simulink model "qrdrls_simulink"  (R2020b)
settings: Solver=FixedStepDiscrete  StartTime=0.0  StopTime=2000  RelTol=1e-3
libraries: dspsrcs4 x2
settings Model: MinMaxOverflowLogging=MinMaxAndOverflow  FPTRunName=NoOverride  Creator=andreas  LastModifiedBy=jgentile
settings DataIOCC: LimitDataPoints=on  SaveFormat=Array  InspectSignalLogs=on  ReturnWorkspaceOutputs=off
settings OptimizationCC: DefaultParameterBehavior=Inlined  ExpressionDepthLimit=2147483647  LifeSpan=inf  SimCompilerOptimization=on
settings DebuggingCC: SignalRangeChecking=warning  UnderspecifiedInitializationDetection=Classic  MergeDetectMultiDrivingBlocksExec=none  SolverPrmCheckMsg=warning  ParameterDowncastMsg=warning  ParameterOverflowMsg=warning  StateNameClashWarn=warning  StrictBusMsg=ErrorOnBusTreatedAsVector  SFUnexpectedBacktrackingDiag=warning  SFNoUnconditionalDefaultTransitionDiag=warning  SFExecutionAtInitializationDiag=none  ArithmeticOperatorsInVariantConditions=warning
settings HardwareCC: ProdBitPerPointer=32  ProdBitPerSizeT=32  ProdBitPerPtrDiffT=32  ProdLargestAtomicFloat=None  ProdIntDivRoundTo=Undefined  ProdEndianess=Unspecified  ProdWordSize=32  ProdHWDeviceType=Generic->Unspecified (assume 32-bit Generic)  TargetBitPerLong=64  TargetBitPerPointer=64  TargetBitPerSizeT=64  TargetBitPerPtrDiffT=64  TargetLongLongMode=on  TargetIntDivRoundTo=Zero  TargetEndianess=LittleEndian  TargetWordSize=64  TargetHWDeviceType=MATLAB Host  ProdEqTarget=off
settings ModelReferenceCC: EnableParallelModelReferenceBuilds=on  PropagateSignalLabelsOutOfModel=off
settings SFSimCC: SimUseLocalCustomCode=off  CustomCodeUndefinedFunction=UseInterfaceOnly
settings RTWCC: RTWUseLocalCustomCode=off
settings CodeAppCC: StateflowObjectComments=on
settings GRTTargetCC: TargetLangStandard=C89/C90 (ANSI)
settings ConfigComp: CovMetricSettings=dw  CovSaveCumulativeToWorkspaceVar=on  CovSaveSingleToWorkspaceVar=on  CovExternalEMLEnable=off

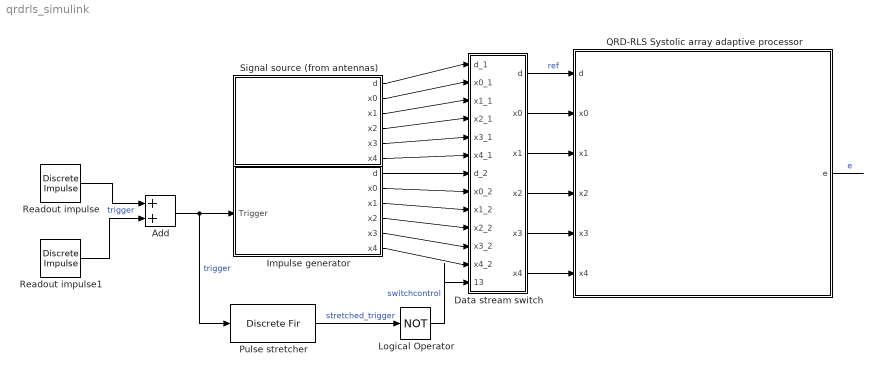
== system qrdrls_simulink ==
  Add : Sum
  Data stream switch : Subsystem
  Impulse generator : Subsystem
  Logical Operator : Logic  Operator=NOT  AllPortsSameDT=off  OutDataTypeStr=boolean
  Pulse stretcher : DiscreteFir  Coefficients=ones(1,6)
  QRD-RLS Systolic array adaptive processor : Subsystem
  Readout impulse : dspsrcs4/Discrete  Impulse  Delay=540  SampleTime=1  FrameSample=1  OutputFrames=on  dataType=double  isSigned=on  wordLen=16  udDataType=sfix(16)  fracBitsMode=Best precision  numFracBits=15  OutDataTypeStr=double  LastOutDataTypeStr=double
  Readout impulse1 : dspsrcs4/Discrete  Impulse  Delay=570  SampleTime=1  FrameSample=1  OutputFrames=on  dataType=double  isSigned=on  wordLen=16  udDataType=sfix(16)  fracBitsMode=Best precision  numFracBits=15  OutDataTypeStr=double  LastOutDataTypeStr=double
  Signal source (from antennas) : Subsystem
  wires:
  QRD-RLS Systolic array adaptive processor/1(e) -> ?  "e"
  Logical Operator/1 -> Data stream switch/13(selector)  "switchcontrol"
  Add/1 -> Pulse stretcher/1, Impulse generator/1(Trigger)  "trigger"
  Signal source (from antennas)/1(d) -> Data stream switch/1(d_1)
  Signal source (from antennas)/2(x0) -> Data stream switch/2(x0_1)
  Signal source (from antennas)/3(x1) -> Data stream switch/3(x1_1)
  Signal source (from antennas)/4(x2) -> Data stream switch/4(x2_1)
  Signal source (from antennas)/5(x3) -> Data stream switch/5(x3_1)
  Signal source (from antennas)/6(x4) -> Data stream switch/6(x4_1)
  Impulse generator/1(d) -> Data stream switch/7(d_2)
  Impulse generator/2(x0) -> Data stream switch/8(x0_2)
  Impulse generator/3(x1) -> Data stream switch/9(x1_2)
  Impulse generator/4(x2) -> Data stream switch/10(x2_2)
  Impulse generator/5(x3) -> Data stream switch/11(x3_2)
  Impulse generator/6(x4) -> Data stream switch/12(x4_2)
  Data stream switch/1(d) -> QRD-RLS Systolic array adaptive processor/1(d)  "ref"
  Data stream switch/2(x0) -> QRD-RLS Systolic array adaptive processor/2(x0)
  Data stream switch/3(x1) -> QRD-RLS Systolic array adaptive processor/3(x1)
  Data stream switch/4(x2) -> QRD-RLS Systolic array adaptive processor/4(x2)
  Data stream switch/5(x3) -> QRD-RLS Systolic array adaptive processor/5(x3)
  Data stream switch/6(x4) -> QRD-RLS Systolic array adaptive processor/6(x4)
  Pulse stretcher/1 -> Logical Operator/1  "stretched_trigger"
  Readout impulse/1 -> Add/1  "trigger"
  Readout impulse1/1 -> Add/2

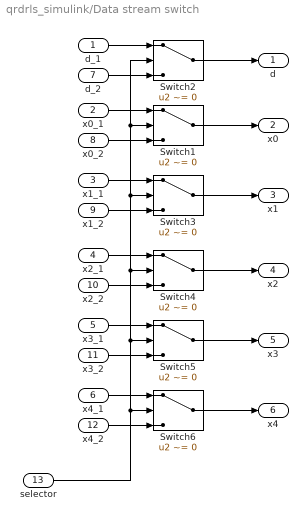
== system qrdrls_simulink/Data stream switch ==
  d_1 : Inport
  x0_1 : Inport  Port=2
  x1_1 : Inport  Port=3
  x2_1 : Inport  Port=4
  x3_1 : Inport  Port=5
  x4_1 : Inport  Port=6
  d_2 : Inport  Port=7
  x0_2 : Inport  Port=8
  x1_2 : Inport  Port=9
  x2_2 : Inport  Port=10
  x3_2 : Inport  Port=11
  x4_2 : Inport  Port=12
  selector : Inport  Port=13
  Switch{1..6} (6 alike) : Switch  Criteria=u2 ~= 0
  d : Outport
  x0 : Outport  Port=2
  x1 : Outport  Port=3
  x2 : Outport  Port=4
  x3 : Outport  Port=5
  x4 : Outport  Port=6
  wires:
  d_1/1 -> Switch2/1
  d_2/1 -> Switch2/3
  Switch2/1 -> d/1
  x0_1/1 -> Switch1/1
  x0_2/1 -> Switch1/3
  x1_1/1 -> Switch3/1
  x1_2/1 -> Switch3/3
  x2_1/1 -> Switch4/1
  x2_2/1 -> Switch4/3
  x3_1/1 -> Switch5/1
  x3_2/1 -> Switch5/3
  x4_1/1 -> Switch6/1
  x4_2/1 -> Switch6/3
  Switch1/1 -> x0/1
  Switch3/1 -> x1/1
  Switch4/1 -> x2/1
  Switch5/1 -> x3/1
  Switch6/1 -> x4/1
  selector/1 -> Switch6/2, Switch5/2, Switch4/2, Switch3/2, Switch1/2, Switch2/2

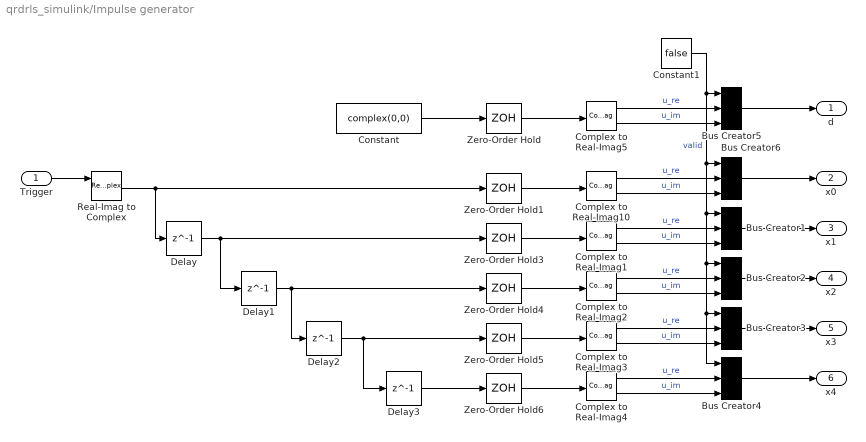
== system qrdrls_simulink/Impulse generator ==
  Trigger : Inport
  Bus Creator{1..6} (6 alike) : BusCreator  Inputs=3  OutDataTypeStr=Bus: vbus  NonVirtualBus=on
  Complex to Real-Imag{1..5,10} (6 alike) : ComplexToRealImag
  Constant : Constant  Value=complex(0,0)
  Constant1 : Constant  Value=false
  Delay{,1..3} (4 alike) : Delay  DelayLength=1  InitialCondition=0
  Real-Imag to Complex : RealImagToComplex
  Zero-Order Hold{,1,3..6} (6 alike) : ZeroOrderHold
  d : Outport
  x0 : Outport  Port=2
  x1 : Outport  Port=3
  x2 : Outport  Port=4
  x3 : Outport  Port=5
  x4 : Outport  Port=6
  wires:
  Delay3/1 -> Zero-Order Hold6/1
  Delay2/1 -> Zero-Order Hold5/1, Delay3/1
  Delay1/1 -> Zero-Order Hold4/1, Delay2/1
  Delay/1 -> Zero-Order Hold3/1, Delay1/1
  Real-Imag to Complex/1 -> Delay/1, Zero-Order Hold1/1
  Constant/1 -> Zero-Order Hold/1
  Trigger/1 -> Real-Imag to Complex/1
  Zero-Order Hold1/1 -> Complex to Real-Imag10/1
  Complex to Real-Imag10/1 -> Bus Creator6/2  "u_re"
  Complex to Real-Imag10/2 -> Bus Creator6/3  "u_im"
  Bus Creator6/1 -> x0/1
  Complex to Real-Imag1/1 -> Bus Creator1/2  "u_re"
  Complex to Real-Imag1/2 -> Bus Creator1/3  "u_im"
  Complex to Real-Imag2/1 -> Bus Creator2/2  "u_re"
  Complex to Real-Imag2/2 -> Bus Creator2/3  "u_im"
  Complex to Real-Imag3/1 -> Bus Creator3/2  "u_re"
  Complex to Real-Imag3/2 -> Bus Creator3/3  "u_im"
  Complex to Real-Imag4/1 -> Bus Creator4/2  "u_re"
  Complex to Real-Imag4/2 -> Bus Creator4/3  "u_im"
  Zero-Order Hold5/1 -> Complex to Real-Imag3/1
  Zero-Order Hold4/1 -> Complex to Real-Imag2/1
  Zero-Order Hold3/1 -> Complex to Real-Imag1/1
  Zero-Order Hold6/1 -> Complex to Real-Imag4/1
  Bus Creator1/1 -> x1/1
  Bus Creator2/1 -> x2/1
  Bus Creator3/1 -> x3/1
  Bus Creator4/1 -> x4/1
  Constant1/1 -> Bus Creator5/1, Bus Creator4/1, Bus Creator3/1, Bus Creator2/1, Bus Creator1/1, Bus Creator6/1  "valid"
  Complex to Real-Imag5/1 -> Bus Creator5/2  "u_re"
  Complex to Real-Imag5/2 -> Bus Creator5/3  "u_im"
  Bus Creator5/1 -> d/1
  Zero-Order Hold/1 -> Complex to Real-Imag5/1

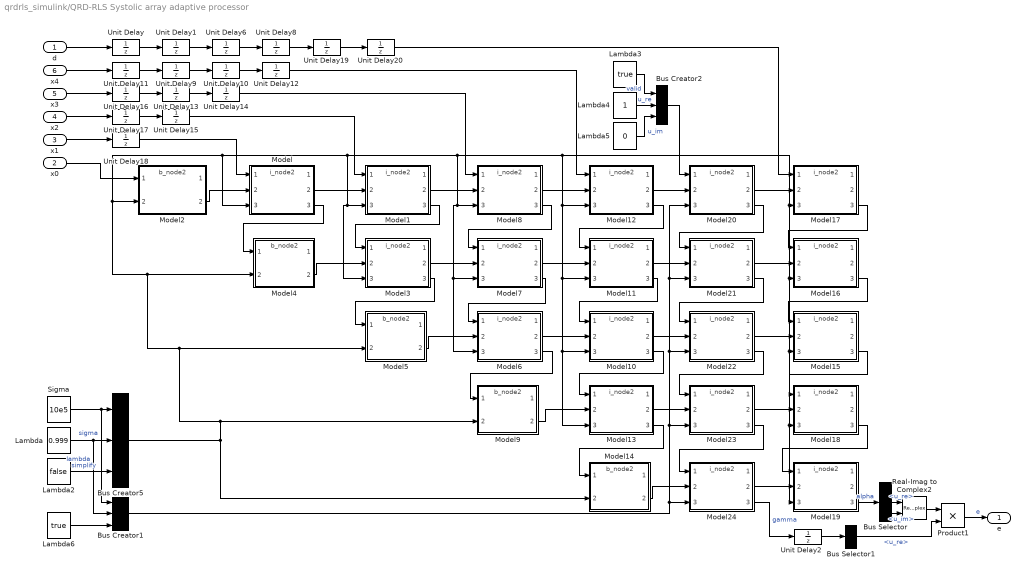
== system qrdrls_simulink/QRD-RLS Systolic array adaptive processor ==
  d : Inport
  x0 : Inport  Port=2
  x1 : Inport  Port=3
  x2 : Inport  Port=4
  x3 : Inport  Port=5
  x4 : Inport  Port=6
  Bus Creator1 : BusCreator  Inputs=3  OutDataTypeStr=Bus: cbus
  Bus Creator2 : BusCreator  Inputs=3
  Bus Creator5 : BusCreator  Inputs=3  OutDataTypeStr=Bus: cbus
  Bus Selector : BusSelector  OutputSignals=valid,u_re,u_im
  Bus Selector1 : BusSelector  OutputSignals=valid,u_re,u_im
  Lambda : Constant  Value=0.999  VectorParams1D=off  OutDataTypeStr=double
  Lambda2 : Constant  Value=false  VectorParams1D=off  OutDataTypeStr=boolean
  Lambda3 : Constant  Value=true  VectorParams1D=off  OutDataTypeStr=boolean
  Lambda4 : Constant  VectorParams1D=off  OutDataTypeStr=double
  Lambda5 : Constant  Value=0  VectorParams1D=off  OutDataTypeStr=double
  Lambda6 : Constant  Value=true  VectorParams1D=off  OutDataTypeStr=boolean
  Model{,1,3,6..8,10..13,15..24} (20 alike) : ModelReference  ModelNameDialog=i_node2  SimulationMode=Normal  ModelReferenceVersion=1.145
  Model{2,4..5,9,14} (5 alike) : ModelReference  ModelNameDialog=b_node2  SimulationMode=Normal  ModelReferenceVersion=1.120
  Product1 : Product  OutDataTypeStr=double  RndMeth=Zero
  Real-Imag to Complex2 : RealImagToComplex
  Sigma : Constant  Value=10e5  VectorParams1D=off  OutDataTypeStr=double
  Unit Delay{,1..2,6,8..20} (17 alike) : UnitDelay  SampleTime=-1  HasFrameUpgradeWarning=on
  e : Outport
  wires:
  Unit Delay19/1 -> Unit Delay20/1
  Bus Creator5/1 -> Model14/2, Model9/2, Model5/2, Model2/2, Model17/3, Model16/3, Model15/3, Model18/3, Model19/3, Model12/3, Model11/3, Model10/3, Model13/3, Model6/3, Model7/3, Model8/3, Model3/3, Model1/3, Model/3, Model4/2
  Sigma/1 -> Bus Creator1/1, Bus Creator5/1  "sigma"
  Lambda/1 -> Bus Creator1/2, Bus Creator5/2  "lambda"
  Bus Selector/3 -> Real-Imag to Complex2/2  "<u_im>"
  Bus Selector/2 -> Real-Imag to Complex2/1  "<u_re>"
  Real-Imag to Complex2/1 -> Product1/1
  Unit Delay/1 -> Unit Delay1/1
  Unit Delay10/1 -> Unit Delay12/1
  Unit Delay9/1 -> Unit Delay10/1
  Unit Delay11/1 -> Unit Delay9/1
  x4/1 -> Unit Delay11/1
  d/1 -> Unit Delay/1
  Unit Delay13/1 -> Unit Delay14/1
  Unit Delay16/1 -> Unit Delay13/1
  x1/1 -> Unit Delay18/1
  Unit Delay15/1 -> Model1/1
  Unit Delay17/1 -> Unit Delay15/1
  x2/1 -> Unit Delay17/1
  x3/1 -> Unit Delay16/1
  x0/1 -> Model2/1
  Unit Delay18/1 -> Model/1
  Unit Delay14/1 -> Model8/1
  Unit Delay12/1 -> Model12/1
  Model2/2 -> Model/2
  Model/2 -> Model1/2
  Model1/2 -> Model8/2
  Model8/2 -> Model12/2
  Model4/2 -> Model3/2
  Model3/2 -> Model7/2
  Model7/2 -> Model11/2
  Model5/2 -> Model6/2
  Model6/2 -> Model10/2
  Model9/2 -> Model13/2
  Model18/3 -> Model19/1
  Model15/3 -> Model18/1
  Model16/3 -> Model15/1
  Model17/3 -> Model16/1
  Model12/3 -> Model11/1
  Model11/3 -> Model10/1
  Model10/3 -> Model13/1
  Model13/3 -> Model14/1
  Model8/3 -> Model7/1
  Model1/3 -> Model3/1
  Model/3 -> Model4/1
  Model3/3 -> Model5/1
  Model7/3 -> Model6/1
  Model6/3 -> Model9/1
  Model19/3 -> Bus Selector/1  "alpha"
  Unit Delay1/1 -> Unit Delay6/1
  Unit Delay6/1 -> Unit Delay8/1
  Unit Delay8/1 -> Unit Delay19/1
  Lambda2/1 -> Bus Creator5/3  "simplify"
  Model12/2 -> Model20/2
  Model11/2 -> Model21/2
  Model10/2 -> Model22/2
  Model13/2 -> Model23/2
  Model14/2 -> Model24/2
  Model20/2 -> Model17/2
  Model21/2 -> Model16/2
  Model22/2 -> Model15/2
  Model23/2 -> Model18/2
  Model24/2 -> Model19/2
  Model20/3 -> Model21/1
  Model21/3 -> Model22/1
  Model22/3 -> Model23/1
  Model23/3 -> Model24/1
  Bus Creator1/1 -> Model23/3, Model22/3, Model21/3, Model20/3, Model24/3
  Lambda4/1 -> Bus Creator2/2  "u_re"
  Bus Creator2/1 -> Model20/1
  Lambda5/1 -> Bus Creator2/3  "u_im"
  Lambda3/1 -> Bus Creator2/1  "valid"
  Bus Selector1/2 -> Product1/2  "<u_re>"
  Model24/3 -> Unit Delay2/1  "gamma"
  Product1/1 -> e/1  "e"
  Lambda6/1 -> Bus Creator1/3
  Unit Delay20/1 -> Model17/1
  Unit Delay2/1 -> Bus Selector1/1

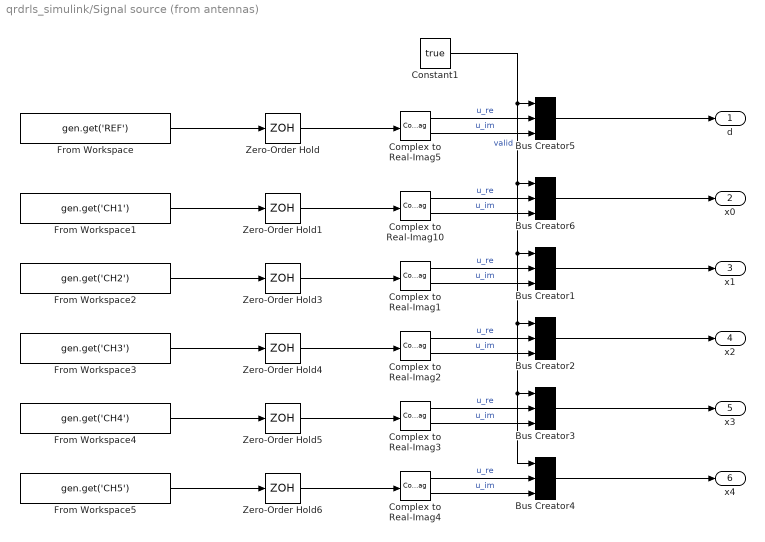
== system qrdrls_simulink/Signal source (from antennas) ==
  Bus Creator{1..6} (6 alike) : BusCreator  Inputs=3  OutDataTypeStr=Bus: vbus  NonVirtualBus=on
  Complex to Real-Imag{1..5,10} (6 alike) : ComplexToRealImag
  Constant1 : Constant  Value=true
  From Workspace : FromWorkspace  VariableName=gen.get('REF')
  From Workspace1 : FromWorkspace  VariableName=gen.get('CH1')
  From Workspace2 : FromWorkspace  VariableName=gen.get('CH2')
  From Workspace3 : FromWorkspace  VariableName=gen.get('CH3')
  From Workspace4 : FromWorkspace  VariableName=gen.get('CH4')
  From Workspace5 : FromWorkspace  VariableName=gen.get('CH5')
  Zero-Order Hold{,1,3..6} (6 alike) : ZeroOrderHold
  d : Outport
  x0 : Outport  Port=2
  x1 : Outport  Port=3
  x2 : Outport  Port=4
  x3 : Outport  Port=5
  x4 : Outport  Port=6
  wires:
  From Workspace/1 -> Zero-Order Hold/1
  From Workspace1/1 -> Zero-Order Hold1/1
  From Workspace2/1 -> Zero-Order Hold3/1
  From Workspace3/1 -> Zero-Order Hold4/1
  From Workspace4/1 -> Zero-Order Hold5/1
  From Workspace5/1 -> Zero-Order Hold6/1
  Zero-Order Hold1/1 -> Complex to Real-Imag10/1
  Zero-Order Hold/1 -> Complex to Real-Imag5/1
  Complex to Real-Imag10/1 -> Bus Creator6/2  "u_re"
  Complex to Real-Imag10/2 -> Bus Creator6/3  "u_im"
  Bus Creator6/1 -> x0/1
  Complex to Real-Imag1/1 -> Bus Creator1/2  "u_re"
  Complex to Real-Imag1/2 -> Bus Creator1/3  "u_im"
  Complex to Real-Imag2/1 -> Bus Creator2/2  "u_re"
  Complex to Real-Imag2/2 -> Bus Creator2/3  "u_im"
  Complex to Real-Imag3/1 -> Bus Creator3/2  "u_re"
  Complex to Real-Imag3/2 -> Bus Creator3/3  "u_im"
  Complex to Real-Imag4/1 -> Bus Creator4/2  "u_re"
  Complex to Real-Imag4/2 -> Bus Creator4/3  "u_im"
  Zero-Order Hold5/1 -> Complex to Real-Imag3/1
  Zero-Order Hold4/1 -> Complex to Real-Imag2/1
  Zero-Order Hold3/1 -> Complex to Real-Imag1/1
  Zero-Order Hold6/1 -> Complex to Real-Imag4/1
  Bus Creator1/1 -> x1/1
  Bus Creator2/1 -> x2/1
  Bus Creator3/1 -> x3/1
  Bus Creator4/1 -> x4/1
  Constant1/1 -> Bus Creator5/1, Bus Creator4/1, Bus Creator3/1, Bus Creator2/1, Bus Creator1/1, Bus Creator6/1  "valid"
  Complex to Real-Imag5/1 -> Bus Creator5/2  "u_re"
  Complex to Real-Imag5/2 -> Bus Creator5/3  "u_im"
  Bus Creator5/1 -> d/1
